simulink model "uz_3ph_ParameterID"  (R2022b)
settings: Solver=FixedStepDiscrete  StartTime=0.0  StopTime=160  FixedStep=0.000005  RelTol=1e-3  EnableMultiTasking=on
model workspace (MATLAB code in the model file):
  | cmdLim = Simulink.Parameter;
  | cmdLim.Value = 15;
  | cmdLim.Description = 'Limit for controlling the maximum surface command angle.';
  | cmdLim.Min = 0;
  | cmdLim.Max = 90;
  | cmdLim.DocUnits = 'deg';
  | 
  | dispGain = Simulink.Parameter;
  | dispGain.Value = 0.75;
  | dispGain.Description = 'Gain applied to the displacement error.';
  | dispGain.Min = 0;
  | dispGain.Max = [];
  | dispGain.DocUnits = 'deg/sec/deg';
  | 
  | dispLim = Simulink.Parameter;
  | dispLim.Value = 30;
  | dispLim.Description = 'Limit for controlling the maximum commanded angle.';
  | dispLim.Min = 0;
  | dispLim.Max = 180;
  | dispLim.DocUnits = 'deg';
  | 
  | intGain = Simulink.Parameter;
  | intGain.Value = 0.5;
  | intGain.Description = 'Gain applied to the integral error.';
  | intGain.Min = 0;
  | intGain.Max = [];
  | intGain.DocUnits = 'deg/sec/deg/sec';
  | 
  | intLim = Simulink.Parameter;
  | intLim.Value = 5;
  | intLim.Description = 'Limit for controlling the maximum commanded angle.';
  | intLim.Min = 0;
  | intLim.Max = 90;
  | intLim.DocUnits = 'deg';
  | 
  | rateGain = Simulink.Parameter;
  | rateGain.Value = 2;
  | rateGain.Description = 'Gain applied to the rate error.';
  | rateGain.Min = 0;
  | rateGain.Max = [];
  | rateGain.DocUnits = 'deg/deg/sec';
  | 
  | rateLim = Simulink.Parameter;
  | rateLim.Value = 6;
  | rateLim.Description = 'Limit for controlling the maximum commanded angle.';
  | rateLim.Min = 0;
  | rateLim.Max = 180;
  | rateLim.DocUnits = 'deg/sec';
  | 
  | hdgGain = Simulink.Parameter;
  | hdgGain.Value = 0.015;
values from neighbouring files (symbols this model uses):
  d_d_TMS = 0.005    [Parameter_Init_Buehler_201.m]
  d_f_hardware = 200000    [Parameter_Init_Buehler_201.m]
  d_f_states = 20000    [Parameter_Init_Buehler_201.m]
  d_i_max = 15    [Parameter_Init_Buehler_201.m]
  d_i_min = -d_i_max    (= -15)    [Parameter_Init_Buehler_201.m]
  d_I_n = 8    [Parameter_Init_Buehler_201.m]
  d_J_Coupling_M_E = 2e-6    (= 2e-06)    [Parameter_Init_Buehler_201.m]
  d_J_Coupling_M_Ms = 2e-20    [Parameter_Init_Buehler_201.m]
  d_J_Ms_L = d_J_Ms_M    (= 1.26363648e-05)    [Parameter_Init_Buehler_201.m]
  d_J_Ms_M = 0.5*0.5*((0.5*d_d_Ms)^4)*3.14*d_l_Ms*d_rho_Ms    (= 1.26363648e-05)    [Parameter_Init_Buehler_201.m]
  d_L_d = 0.00031    [Parameter_Init_Buehler_201.m]
  d_L_q = 0.00033    [Parameter_Init_Buehler_201.m]
  d_p = 4    [Parameter_Init_Buehler_201.m]
  d_psi_pm = 0.0075    [Parameter_Init_Buehler_201.m]
  d_R_ph = d_R_ph_ph/2    (= 0.089)    [Parameter_Init_Buehler_201.m]
  d_y_max = 10    [Parameter_Init_Buehler_201.m]
  d_y_min = -d_y_max    (= -10)    [Parameter_Init_Buehler_201.m]
undefined symbols (not defined in the file or in its folder): i_dq, i_dq_ref, n_ref, V_abc, v_dq
libraries: fl_lib x47, nesl_utility x30, ee_lib x18, simulink x8, spsabctodq0Lib x2, spsdq0toabcLib x1, spsTriangleGeneratorLib x1
(part 4 of 4)

== matlab function uz_3ph_ParameterID/FOC/Space vector limitation ==
  data: v_d_limit output; v_q_limit output; ActualValues input; v_d_in input single; v_q_in input; limit_on output boolean
% Algorithm for voltage space vector limitation
% 
% Quelle:    Vector Control of Three-Phase AC Machines, S. 183
% Autoren:   Nguyen Phung Quang, Jörg-Andreas Dittrich
%            Springer, 2015,Second Edition


function [v_d_limit, v_q_limit,limit_on] = fcn(ActualValues,v_d_in, v_q_in)
% max amplitude of the space vectors
   % with addition of 3rd harmonics   U^_LN = V_DC/2;
   %V_DC_max = V_DC*0.5;
   %with offset addition of 3rd harmonics  V^_LN = V_DC/sqrt(3);
   V_SV_max =ActualValues.V_DC/sqrt(3);

% absolue value of the space vector from vd and vq
V_SV_abs = sqrt(v_d_in^2 + v_q_in^2);

% limitation necessary?
if ( V_SV_abs > V_SV_max )   
    limit_on = boolean(1);   % limitation is necessary -> generator or drive operation?
   
    if ((sign(ActualValues.omega_el)==sign(ActualValues.i_dq.q)) ) % drive operation      
        Error = 0;
        if ( (abs(v_d_in) > 0.95*V_SV_max) )
        %true
        v_d_limit = sign(v_d_in)*0.95*V_SV_max;
        v_q_limit = sign(v_q_in)*sqrt(V_SV_max^2-v_d_limit^2);
        Fall = 2;
        else
        %false
        v_d_limit = v_d_in;
        v_q_limit = sign(v_q_in)*sqrt(V_SV_max^2-v_d_limit^2);
        Fall = 1;
        end    
    
    
    elseif ((sign(ActualValues.omega_el)~=sign(ActualValues.i_dq.q)) ) % generator operation   
        Error = 0;
        if ( abs(v_q_in) > 0.95*V_SV_max )
        %true
        v_q_limit = sign(v_q_in)*0.95*V_SV_max;
        v_d_limit = sign(v_d_in)*sqrt(V_SV_max^2-v_q_limit^2);
        %v_d_limit = U_d;        Fall = 4;       
        else 
        % false
        v_q_limit = v_q_in;
        v_d_limit = sign(v_d_in)*sqrt(V_SV_max^2-v_q_limit^2);
        Fall = 3;
        end
        
    else % Error
    v_d_limit = v_d_in;
    v_q_limit = v_q_in;
    Error = 1;
    Fall = 5;
    end
    
else
% no limitation necessary
    v_d_limit = v_d_in;
    v_q_limit = v_q_in;
    limit_on = boolean(0);
    Error = 0;
    Fall = 0;
end

v_d_in = v_d_limit;
v_q_in = v_q_limit;
end

== matlab function uz_3ph_ParameterID/Hardware/12bit ADC1 ==
  data: u input; y output
function y = fcn(u)
%#codegen

y = u*2048/5;

== matlab function uz_3ph_ParameterID/Hardware/12bit ADC ==
  data: u input; y output
function y = fcn(u)
%#codegen

y = u*2048/5;

== matlab function uz_3ph_ParameterID/Hardware/12bit ADC2 ==
  data: u input; y output
function y = fcn(u)
%#codegen

y = u*2048/5;

== matlab function uz_3ph_ParameterID/FOC/Busselector ==
  data: ControlFlags input Bus: uz_ParaID_ControlFlags_t; FOC_state_outputs output Bus: uz_ParaID_Controller_Parameters_output_t; ElectricalID_FOC_input input Bus: uz_ParaID_Controller_Parameters_output_t; FrictionID_FOC_input input Bus: uz_ParaID_Controller_Parameters_output_t; FluxMapID_FOC_input input Bus: uz_ParaID_Controller_Parameters_output_t; TwoMassID_FOC_input input Bus: uz_ParaID_Controller_Parameters_output_t; FOCControl_input input Bus: uz_ParaID_Controller_Parameters_output_t
function FOC_state_outputs = fcn(ControlFlags,ElectricalID_FOC_input,....
    FrictionID_FOC_input,FluxMapID_FOC_input,TwoMassID_FOC_input,FOCControl_input)

switch ControlFlags.transNr
    case 0
        if(ControlFlags.finished_all_Offline_states==1)
            FOC_state_outputs           = FOCControl_input;
        else
        FOC_state_outputs.i_dq_ref.d          = single(0);
        FOC_state_outputs.i_dq_ref.q          = single(0);
        FOC_state_outputs.i_dq_ref.zero       = single(0);
        FOC_state_outputs.M_ref_FOC           = single(0);
        FOC_state_outputs.activeState         = uint16(0);
        FOC_state_outputs.n_ref_FOC           = single(0);
        FOC_state_outputs.enableFOC_torque    = boolean(0);
        FOC_state_outputs.enableFOC_speed     = boolean(0);
        FOC_state_outputs.enableFOC_current   = boolean(0);
        FOC_state_outputs.resetIntegrator     = boolean(0);
        FOC_state_outputs.Kp_id_out           = single(0);
        FOC_state_outputs.Kp_iq_out           = single(0);
        FOC_state_outputs.Kp_n_out            = single(0);
        FOC_state_outputs.Ki_id_out           = single(0);
        FOC_state_outputs.Ki_iq_out           = single(0);
        FOC_state_outputs.Ki_n_out            = single(0);
        end
    case 1
        FOC_state_outputs           = ElectricalID_FOC_input;
    case 2
        FOC_state_outputs           = TwoMassID_FOC_input;
    case 3
        FOC_state_outputs           = FrictionID_FOC_input;
    case 4
        FOC_state_outputs           = FluxMapID_FOC_input;
    otherwise
        FOC_state_outputs.i_dq_ref.d          = single(0);
        FOC_state_outputs.i_dq_ref.q          = single(0);
        FOC_state_outputs.i_dq_ref.zero       = single(0);
        FOC_state_outputs.M_ref_FOC           = single(0);
        FOC_state_outputs.activeState         = uint16(0);
        FOC_state_outputs.n_ref_FOC           = single(0);
        FOC_state_outputs.enableFOC_torque    = boolean(0);
        FOC_state_outputs.enableFOC_speed     = boolean(0);
        FOC_state_outputs.enableFOC_current   = boolean(0);
        FOC_state_outputs.resetIntegrator     = boolean(0);
        FOC_state_outputs.Kp_id_out           = single(0);
        FOC_state_outputs.Kp_iq_out           = single(0);
        FOC_state_outputs.Kp_n_out            = single(0);
        FOC_state_outputs.Ki_id_out           = single(0);
        FOC_state_outputs.Ki_iq_out           = single(0);
        FOC_state_outputs.Ki_n_out            = single(0);
end
        FOC_state_outputs.i_xy_ref.d          = single(0);
        FOC_state_outputs.i_xy_ref.q          = single(0);
        FOC_state_outputs.i_xy_ref.zero       = single(0);
        FOC_state_outputs.i_zero_ref.d          = single(0);
        FOC_state_outputs.i_zero_ref.q          = single(0);
        FOC_state_outputs.i_zero_ref.zero       = single(0);
        FOC_state_outputs.PI_dq                 = boolean(0);
        FOC_state_outputs.PI_xy                 = boolean(0);
        FOC_state_outputs.PI_zero               = boolean(0);
        FOC_state_outputs.resonant_dq           = boolean(0);
        FOC_state_outputs.resonant_xy           = boolean(0);
        FOC_state_outputs.resonant_zero         = boolean(0);
        FOC_state_outputs.filter_dq             = boolean(0);
        FOC_state_outputs.filter_xy             = boolean(0);
        FOC_state_outputs.filter_zero           = boolean(0);
end

== matlab function uz_3ph_ParameterID/InterpMeshGrid ==
  data: FluxMapData output Bus: uz_ParaID_FluxMapsData_t; psi_array_in input; i_rat input; OnlineID_input input
function FluxMapData = fcn(psi_array_in,i_rat,OnlineID_input)
%Author Philipp Gebhardt
% Oktober 2019

%This function is calculating the regular flux maps out of the irregular scatter data array stored in psi_array_in. The Outputs rangeX are containg the flux maps axis information which range is related to 3 times i_rat input.
%Furthermore the temperature dependency of the permanent flux is calculated if there are enough measuring values stored in the delta_psi_array. The temperature constant as well as the estimated error of permanent flux
%at reference temperature are given out on psi_temp_const and psi_temp_error outputs.  Using this temperature dependency the flux maps are updated with the permanent flux offset caused by the temperature which is given
%in on OnlineID_input.Wtemp input. 

%-----------------------------------------------------------------------------------------------------------------------------------------
%initalising Outputs
%-----------------------------------------------------------------------------------------------------------------------------------------

psi_array=zeros(6,100);
psi_array=psi_array_in;
delta_psi=zeros(100,1);

FluxMapData.psid_grid=single(zeros(20,20));
FluxMapData.psiq_grid=single(zeros(20,20));
FluxMapData.id_grid=single(zeros(20,20));
FluxMapData.iq_grid=single(zeros(20,20));
FluxMapData.range_id_Y=single(zeros(1,20));
FluxMapData.range_psid_Y=single(zeros(1,20));
FluxMapData.range_psiq_Y=single(zeros(1,20));
FluxMapData.range_psid_X=single(zeros(1,20));
FluxMapData.range_psiq_X=single(zeros(1,20));
FluxMapData.range_iq_Y=single(zeros(1,20));
FluxMapData.range_iq_X=single(zeros(1,20));
FluxMapData.range_id_X=single(zeros(1,20));
FluxMapData.psi_temp_const=single(0.000001);
FluxMapData.psi_temp_error=single(0);



range_psid_X_in=single(zeros(1,20));
range_psid_Y_in=single(zeros(1,20));
range_psiq_X_in=single(zeros(1,20));
range_psiq_Y_in=single(zeros(1,20));
range_id_X_in=single(zeros(1,20));
range_id_Y_in=single(zeros(1,20));
range_iq_X_in=single(zeros(1,20));
range_iq_Y_in=single(zeros(1,20));


%initalise range of flux maps axis
for t=single(0):single(19)
   range_psid_X_in(t+1)=-3*i_rat+t*4*i_rat/19;
   range_psid_Y_in(t+1)=-3*i_rat+t*6*i_rat/19;
   range_psiq_X_in(t+1)=-3*i_rat+t*4*i_rat/19;
   range_psiq_Y_in(t+1)=-3*i_rat+t*6*i_rat/19;
end

%Calculate flux deviation from amout of measuring values and counter sum,
%to average a big amount of measuring values 

for t=single(1):single(100)
    if (OnlineID_input.delta_psi(t,2)>5)
    delta_psi(t,1)=OnlineID_input.delta_psi(t,1)/OnlineID_input.delta_psi(t,2);
    end
end

%Calculate temperature constant with a regressionline, set second input "1"
%to resist outliers greater than 30% (relative to their neighbours)

[psi_temp_const_test,FluxMapData.psi_temp_error]=regressionline(delta_psi,1);

%check plausibility
if(psi_temp_const_test>0&&FluxMapData.psi_temp_const<10)%in mVs/°C
FluxMapData.psi_temp_const=psi_temp_const_test;
end


%correct temperature offset
 for k=single(1):single(100)
   if(psi_array(3,k)~=0)
    psi_array(5,k)=psi_array(5,k)+(psi_array(4,k)-OnlineID_input.Wtemp)*FluxMapData.psi_temp_const;
    psi_array(4,k)=OnlineID_input.Wtemp;
   end
end





%Inter- and extrapolation of the flux maps 
[FluxMapData.range_psid_X,FluxMapData.range_psid_Y,FluxMapData.psid_grid] = interpol_flux_scatter_psid ([psi_array(1,:);psi_array(2,:);psi_array(5,:);zeros(length(psi_array(1,:)))],range_psid_X_in,range_psid_Y_in);
[FluxMapData.range_psiq_X,FluxMapData.range_psiq_Y,FluxMapData.psiq_grid] = interpol_flux_scatter_psiq ([psi_array(1,:);psi_array(2,:);psi_array(6,:);zeros(length(psi_array(1,:)))],range_psiq_X_in,range_psiq_Y_in);

%initialise range of inverse flux maps axis
for t=single(0):single(19)
   range_id_X_in(t+1)=min(min(FluxMapData.psid_grid))+t*(max(max(FluxMapData.psid_grid))-min(min(FluxMapData.psid_grid)))/19;
   range_id_Y_in(t+1)=min(min(FluxMapData.psiq_grid))+t*(max(max(FluxMapData.psiq_grid))-min(min(FluxMapData.psiq_grid)))/19;
   range_iq_X_in(t+1)=min(min(FluxMapData.psid_grid))+t*(max(max(FluxMapData.psid_grid))-min(min(FluxMapData.psid_grid)))/19;
   range_iq_Y_in(t+1)=min(min(FluxMapData.psiq_grid))+t*(max(max(FluxMapData.psiq_grid))-min(min(FluxMapData.psiq_grid)))/19;
end

%Inter and extrapolate inverse flux maps
[FluxMapData.range_id_X,FluxMapData.range_id_Y,FluxMapData.id_grid] = interpol_flux_scatter_psid ([psi_array(5,:);psi_array(6,:);psi_array(1,:);zeros(length(psi_array(1,:)))],range_id_X_in,range_id_Y_in);
[FluxMapData.range_iq_X,FluxMapData.range_iq_Y,FluxMapData.iq_grid] = interpol_flux_scatter_psiq ([psi_array(5,:);psi_array(6,:);psi_array(2,:);zeros(length(psi_array(1,:)))],range_iq_X_in,range_iq_Y_in);

end

== stateflow chart uz_3ph_ParameterID/AutoRefCurrents ==
  settings: updateMethod=DISCRETE  sampleTime=1/d_f_states
  note: Philipp Gebhardt, October2019:
      |
      | Description of Control Reference Stateflow:
      |
      | This Stateflow chart is used to generate an cyclic current reference input of d- and q- current. The combinations are circularly arranged in the radius of imax_in.
      | The inputs niq and nid are the amount of measuring values in q- and d-current axis. The input speed_in is used to automatically control the sign of q-current to avoid
      | regenerative current feedback into the inverter.
  state waitState
    entry:
    %do nothing
    %wait for start
  state superstate
    entry:
    counter=single(19998);
    %counter=single(17498);
    iqcount=single(0);
    idcount=single(-AutoRefCurrentsConfig.id_points/3);
    AutoRefCurrents_state_output.i_dq_ref.d=single(0);
    AutoRefCurrents_state_output.i_dq_ref.q=single(0);
    imax=single(0);
    state stepstate
      entry:
      if(ActualValues.omega_m>0)
      imax=abs(AutoRefCurrentsConfig.max_current);
      end
      if(ActualValues.omega_m<0)
      imax=abs(AutoRefCurrentsConfig.max_current)*-1;
      end
      if((AutoRefCurrents_state_output.i_dq_ref.d*AutoRefCurrents_state_output.i_dq_ref.d+(imax*iqcount/AutoRefCurrentsConfig.iq_points)^2)^0.5<abs(imax))
      AutoRefCurrents_state_output.i_dq_ref.q=imax*iqcount/AutoRefCurrentsConfig.iq_points;
      else
      iqcount=single(1);
      AutoRefCurrents_state_output.i_dq_ref.q=imax*iqcount/AutoRefCurrentsConfig.iq_points;
      end
      if((AutoRefCurrents_state_output.i_dq_ref.q*AutoRefCurrents_state_output.i_dq_ref.q+(imax*idcount/AutoRefCurrentsConfig.id_points)^2)^0.5<abs(imax))
      AutoRefCurrents_state_output.i_dq_ref.d=-1*abs(imax)*idcount/AutoRefCurrentsConfig.id_points;
      else
      idcount=single(-AutoRefCurrentsConfig.id_points/3);
      AutoRefCurrents_state_output.i_dq_ref.d=-1*abs(imax)*idcount/AutoRefCurrentsConfig.id_points;
      end
      counter=single(0);
    state countstate
      entry:
      if(iqcount<AutoRefCurrentsConfig.iq_points)
      iqcount=iqcount+1;
      else
      iqcount=single(0);
      end
      if(idcount<AutoRefCurrentsConfig.id_points)
      idcount=idcount+1;
      else
      idcount=single(-AutoRefCurrentsConfig.id_points/3);
      end
      during:
      counter=counter+1;
    (default) -> countstate
    countstate -> stepstate : [counter==(2.0/GlobalConfig.sampleTimeISR)]
    stepstate -> countstate : [counter==0]
  (default) -> waitState
  waitState -> superstate : [AutoRefCurrentsConfig.enableCRS==1 &&....
      | AutoRefCurrentsConfig.Reset==0 &&....
      |  GlobalConfig.Reset==0 && GlobalConfig.ACCEPT==1&& ....
      | ControlFlags.finished_all_Offline_states==1]
  superstate -> waitState : [AutoRefCurrentsConfig.enableCRS==0 ||....
      |  AutoRefCurrentsConfig.Reset == 1 ||....
      | GlobalConfig.Reset==1]
      | {AutoRefCurrents_state_output.i_dq_ref.d=single(0);
      | AutoRefCurrents_state_output.i_dq_ref.q=single(0)}
  data: iqcount local; idcount local; counter local; ActualValues input Bus: uz_ParaID_ActualValues_t; imax local; GlobalConfig input Bus: uz_ParaID_GlobalConfig_t; AutoRefCurrentsConfig input Bus: uz_ParaID_AutoRefCurrentsConfig_t; AutoRefCurrents_state_output output Bus: uz_ParaID_AutoRefCurrents_output_t; ControlFlags input Bus: uz_ParaID_ControlFlags_t
